simulink model "labFinal_4"  (R2018b)
settings: Solver=FixedStepDiscrete  StartTime=0.0  StopTime=10.0  FixedStep=1  RelTol=1e-3
libraries: hdlsllib x17
settings Model: Creator=mllax8  LastModifiedBy=mllax8

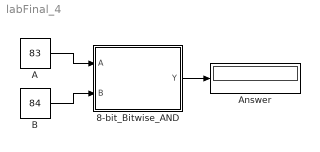
== system labFinal_4 ==
  8-bit_Bitwise_AND : Subsystem
  A : Constant  Value=83  OutDataTypeStr=uint8  SampleTime=1
  Answer : Display
  B : Constant  Value=84  OutDataTypeStr=uint8  SampleTime=1
  wires:
  B/1 -> 8-bit_Bitwise_AND/2(B)
  A/1 -> 8-bit_Bitwise_AND/1(A)
  8-bit_Bitwise_AND/1(Y) -> Answer/1

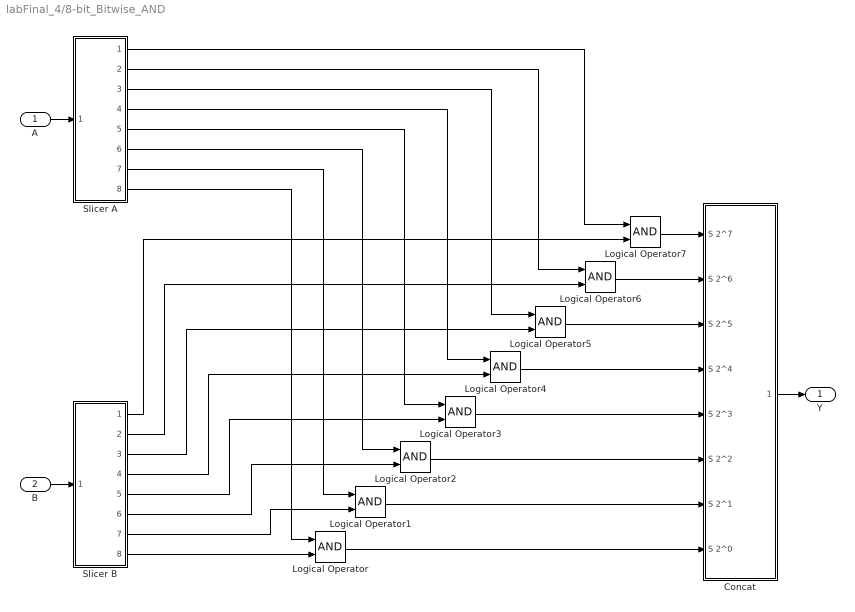
== system labFinal_4/8-bit_Bitwise_AND ==
  A : Inport  OutDataTypeStr=uint8
  B : Inport  Port=2  OutDataTypeStr=uint8
  Concat : Subsystem
  Logical Operator{,1..7} (8 alike) : Logic  AllPortsSameDT=off  OutDataTypeStr=boolean
  Slicer A : Subsystem
  Slicer B : Subsystem
  Y : Outport
  wires:
  B/1 -> Slicer B/1(uint8)
  A/1 -> Slicer A/1(uint8)
  Logical Operator/1 -> Concat/8(S 2^0)
  Slicer B/8("B 2^0 ") -> Logical Operator/2
  Slicer A/8("A 2^0 ") -> Logical Operator/1
  Logical Operator1/1 -> Concat/7(S 2^1)
  Logical Operator2/1 -> Concat/6(S 2^2)
  Logical Operator4/1 -> Concat/4(S 2^4)
  Logical Operator3/1 -> Concat/5(S 2^3)
  Logical Operator5/1 -> Concat/3(S 2^5)
  Logical Operator6/1 -> Concat/2(S 2^6)
  Logical Operator7/1 -> Concat/1(S 2^7)
  Slicer B/7(B 2^1) -> Logical Operator1/2
  Slicer B/6(B 2^2) -> Logical Operator2/2
  Slicer B/5(B 2^3) -> Logical Operator3/2
  Slicer B/4(B 2^4) -> Logical Operator4/2
  Slicer B/3(B 2^5) -> Logical Operator5/2
  Slicer B/2(B 2^6) -> Logical Operator6/2
  Slicer B/1(B 2^7) -> Logical Operator7/2
  Slicer A/7(A 2^1) -> Logical Operator1/1
  Slicer A/6(A 2^2) -> Logical Operator2/1
  Slicer A/5(A 2^3) -> Logical Operator3/1
  Slicer A/4(A 2^4) -> Logical Operator4/1
  Slicer A/3(A 2^5) -> Logical Operator5/1
  Slicer A/2(A 2^6) -> Logical Operator6/1
  Slicer A/1(A 2^7) -> Logical Operator7/1
  Concat/1(unsign Int) -> Y/1

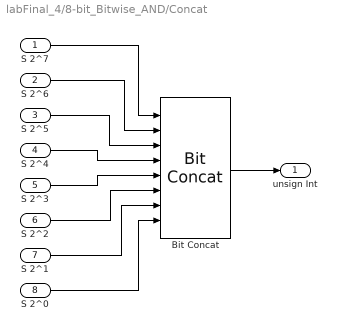
== system labFinal_4/8-bit_Bitwise_AND/Concat ==
  S 2^7 : Inport
  S 2^6 : Inport  Port=2
  S 2^5 : Inport  Port=3
  S 2^4 : Inport  Port=4
  S 2^3 : Inport  Port=5
  S 2^2 : Inport  Port=6
  S 2^1 : Inport  Port=7
  S 2^0 : Inport  Port=8
  Bit Concat : hdlsllib/Logic and Bit Operations/Bit Concat  numInputs=8
      settings: SourceProductName=HDL Coder  SourceProductBaseCode=HD
  unsign Int : Outport
  wires:
  Bit Concat/1 -> unsign Int/1
  S 2^3/1 -> Bit Concat/5
  S 2^5/1 -> Bit Concat/3
  S 2^4/1 -> Bit Concat/4
  S 2^0/1 -> Bit Concat/8
  S 2^7/1 -> Bit Concat/1
  S 2^1/1 -> Bit Concat/7
  S 2^6/1 -> Bit Concat/2
  S 2^2/1 -> Bit Concat/6

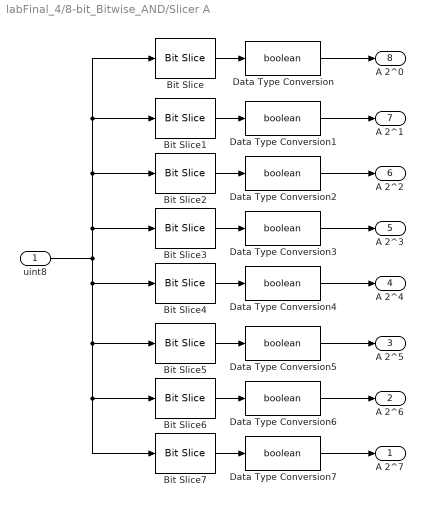
== system labFinal_4/8-bit_Bitwise_AND/Slicer A ==
  uint8 : Inport  OutDataTypeStr=uint8  SampleTime=1
  Bit Slice : hdlsllib/Logic and Bit Operations/Bit Slice  lidx=0  ridx=0
  Bit Slice1 : hdlsllib/Logic and Bit Operations/Bit Slice  lidx=1  ridx=1
  Bit Slice2 : hdlsllib/Logic and Bit Operations/Bit Slice  lidx=2  ridx=2
  Bit Slice3 : hdlsllib/Logic and Bit Operations/Bit Slice  lidx=3  ridx=3
  Bit Slice4 : hdlsllib/Logic and Bit Operations/Bit Slice  lidx=4  ridx=4
  Bit Slice5 : hdlsllib/Logic and Bit Operations/Bit Slice  lidx=5  ridx=5
  Bit Slice6 : hdlsllib/Logic and Bit Operations/Bit Slice  lidx=6  ridx=6
  Bit Slice7 : hdlsllib/Logic and Bit Operations/Bit Slice  lidx=7  ridx=7
  Data Type Conversion{,1..7} (8 alike) : DataTypeConversion  OutDataTypeStr=boolean
  A 2^7 : Outport
  A 2^6 : Outport  Port=2
  A 2^5 : Outport  Port=3
  A 2^4 : Outport  Port=4
  A 2^3 : Outport  Port=5
  A 2^2 : Outport  Port=6
  A 2^1 : Outport  Port=7
  "A 2^0 " : Outport  Port=8
  wires:
  Data Type Conversion/1 -> "A 2^0 "/1
  Data Type Conversion5/1 -> A 2^5/1
  Bit Slice1/1 -> Data Type Conversion1/1
  Bit Slice5/1 -> Data Type Conversion5/1
  Bit Slice7/1 -> Data Type Conversion7/1
  Bit Slice2/1 -> Data Type Conversion2/1
  Bit Slice3/1 -> Data Type Conversion3/1
  Data Type Conversion6/1 -> A 2^6/1
  Bit Slice4/1 -> Data Type Conversion4/1
  uint8/1 -> Bit Slice4/1, Bit Slice5/1, Bit Slice6/1, Bit Slice7/1, Bit Slice3/1, Bit Slice2/1, Bit Slice1/1, Bit Slice/1
  Data Type Conversion1/1 -> A 2^1/1
  Data Type Conversion2/1 -> A 2^2/1
  Bit Slice/1 -> Data Type Conversion/1
  Bit Slice6/1 -> Data Type Conversion6/1
  Data Type Conversion3/1 -> A 2^3/1
  Data Type Conversion4/1 -> A 2^4/1
  Data Type Conversion7/1 -> A 2^7/1

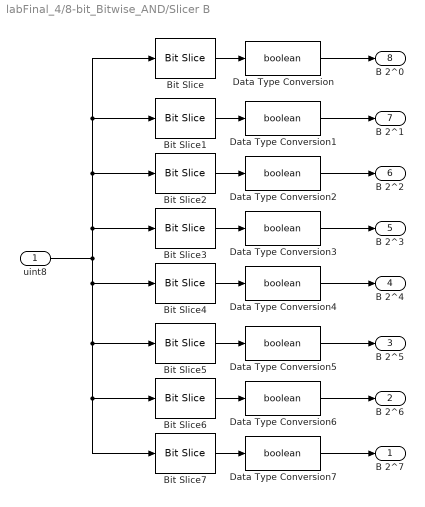
== system labFinal_4/8-bit_Bitwise_AND/Slicer B ==
  uint8 : Inport  OutDataTypeStr=uint8  SampleTime=1
  Bit Slice : hdlsllib/Logic and Bit Operations/Bit Slice  lidx=0  ridx=0
  Bit Slice1 : hdlsllib/Logic and Bit Operations/Bit Slice  lidx=1  ridx=1
  Bit Slice2 : hdlsllib/Logic and Bit Operations/Bit Slice  lidx=2  ridx=2
  Bit Slice3 : hdlsllib/Logic and Bit Operations/Bit Slice  lidx=3  ridx=3
  Bit Slice4 : hdlsllib/Logic and Bit Operations/Bit Slice  lidx=4  ridx=4
  Bit Slice5 : hdlsllib/Logic and Bit Operations/Bit Slice  lidx=5  ridx=5
  Bit Slice6 : hdlsllib/Logic and Bit Operations/Bit Slice  lidx=6  ridx=6
  Bit Slice7 : hdlsllib/Logic and Bit Operations/Bit Slice  lidx=7  ridx=7
  Data Type Conversion{,1..7} (8 alike) : DataTypeConversion  OutDataTypeStr=boolean
  B 2^7 : Outport
  B 2^6 : Outport  Port=2
  B 2^5 : Outport  Port=3
  B 2^4 : Outport  Port=4
  B 2^3 : Outport  Port=5
  B 2^2 : Outport  Port=6
  B 2^1 : Outport  Port=7
  "B 2^0 " : Outport  Port=8
  wires:
  Data Type Conversion/1 -> "B 2^0 "/1
  Data Type Conversion5/1 -> B 2^5/1
  Bit Slice1/1 -> Data Type Conversion1/1
  Bit Slice5/1 -> Data Type Conversion5/1
  Bit Slice7/1 -> Data Type Conversion7/1
  Bit Slice2/1 -> Data Type Conversion2/1
  Bit Slice3/1 -> Data Type Conversion3/1
  Data Type Conversion6/1 -> B 2^6/1
  Bit Slice4/1 -> Data Type Conversion4/1
  uint8/1 -> Bit Slice4/1, Bit Slice5/1, Bit Slice6/1, Bit Slice7/1, Bit Slice3/1, Bit Slice2/1, Bit Slice1/1, Bit Slice/1
  Data Type Conversion1/1 -> B 2^1/1
  Data Type Conversion2/1 -> B 2^2/1
  Bit Slice/1 -> Data Type Conversion/1
  Bit Slice6/1 -> Data Type Conversion6/1
  Data Type Conversion3/1 -> B 2^3/1
  Data Type Conversion4/1 -> B 2^4/1
  Data Type Conversion7/1 -> B 2^7/1
